simulink model "chinasim"  (R2018a)
settings: Solver=FixedStepDiscrete  StartTime=0.0  StopTime=10.0  RelTol=1e-3
InitFcn:
  | mbd_pnt_consistency_checks(bdroot(gcs));
  | t = 1
  | f = 1/t
undefined symbols (not defined in the file): B14, C10
libraries: mbd_pnt_ec_toolbox x4, dspswit3 x1
settings Model: Creator=oolonthegreat  LastModifiedBy=oolonthegreat
settings DataIOCC: ExternalInput=off  InitialState=off  SaveOutput=off  SignalLogging=off  SaveTime=off
settings OptimizationCC: DefaultParameterBehavior=Inlined  EnhancedBackFolding=on  PassReuseOutputArgsAs=Individual arguments  OptimizeBlockOrder=speed  DifferentSizesBufferReuse=on  OptimizationCustomize=off
settings DebuggingCC: InheritedTsInSrcMsg=none  SingleTaskRateTransMsg=error  ParameterTunabilityLossMsg=error  UnconnectedInputMsg=error  UnconnectedOutputMsg=error  UnconnectedLineMsg=error  UnknownTsInhSupMsg=error
settings HardwareCC: ProdBitPerPointer=32  ProdBitPerSizeT=32  ProdBitPerPtrDiffT=32  ProdLargestAtomicInteger=Long  ProdLargestAtomicFloat=Double  ProdEndianess=BigEndian  ProdWordSize=32  ProdHWDeviceType=Motorola PowerPC
settings SFSimCC: MATLABDynamicMemAlloc=off
settings RTWCC: SystemTargetFile=mbd_pnt.tlc  MakeCommand=mbd_pnt_make_rtw COPY_MDLREF_INCLUDES=0  TemplateMakefile=mbd_pnt.tmf  PostCodeGenCommand=mbd_pnt_analyzegencode(buildInfo)  Description=Model Based Design Toolbox MPC574xP Code Generation Target  GenerateReport=on  IncludeHyperlinkInReport=on  LaunchReport=on  GenerateTraceInfo=on  GenerateTraceReport=on  GenerateTraceReportSl=on  GenerateTraceReportSf=on  GenerateTraceReportEml=on
settings CodeAppCC: ForceParamTrailComments=on  IgnoreCustomStorageClasses=off  OperatorAnnotations=on  SimulinkDataObjDesc=on  SFDataObjDesc=on  InsertBlockDesc=on
settings STFCustomTargetCC: TargetLangStandard=C99 (ISO)  MultiwordLength=256  CombineOutputUpdateFcns=on  SuppressErrorStatus=on  ERTCustomFileBanners=on  SupportContinuousTime=off  SupportNonInlinedSFcns=off  RemoveResetFunc=on  MATLABClassNameForMDSCustomization=Simulink.SoftwareTarget.ERTCustomization  GRTInterface=off  SystemTargetFile=mbd_pnt.tlc
settings ERTTargetCC: TargetLangStandard=C99 (ISO)  ParMdlRefBuildCompliant=off  CompOptLevelCompliant=off  ConcurrentExecutionCompliant=off  SuppressErrorStatus=on  ModelStepFunctionPrototypeControlCompliant=off  CPPClassGenCompliant=off  UseToolchainInfoCompliant=off  InlinedParameterPlacement=NonHierarchical  ERTCustomFileTemplate=example_file_process.tlc

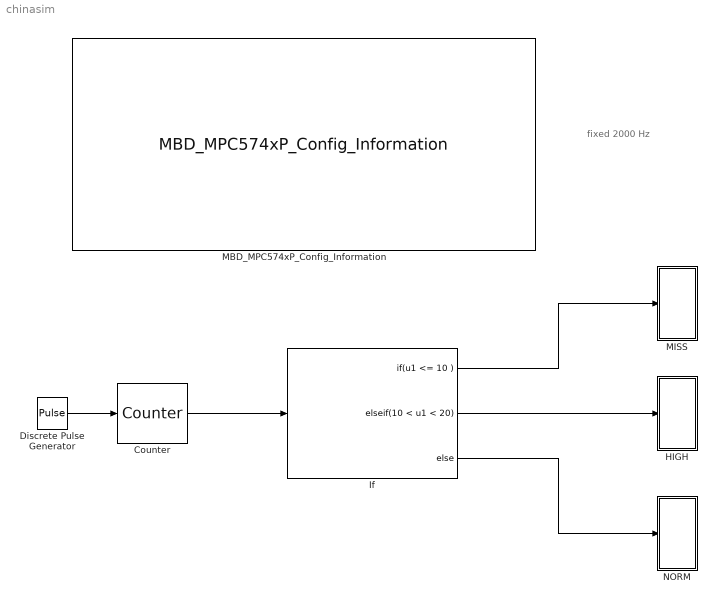
== system chinasim ==
  note: fixed 2000 Hz
  Counter : dspswit3/Counter  Direction=Up  CountEvent=Rising edge  CounterSize=User defined  MaxCount=40  InitialCount=1  Output=Count  HitValue=32  ResetInput=off  SamplesPerFrame=1  Ts=1  CntDtype=double  HitDtype=Logical
  Discrete Pulse Generator : DiscretePulseGenerator  Period=100  PulseWidth=50  SampleTime=t/10
  HIGH : Subsystem  TreatAsAtomicUnit=on
  If : If  IfExpression=u1 <= 10  ElseIfExpressions=10 < u1 < 20
  MBD_MPC574xP_Config_Information : mbd_pnt_ec_toolbox/MPC574xP/MBD_MPC574xP_Config_Information  disp_str=|  config_params=[]
      | System Clock : 200 MHz
      | Target : MPC5744P
      | Package : 144LQFP
      | XTAL Freq : 40 MHz
      | Compiler : S32 Design Studio
      | Target Type : FLASH
      | Global Interrupt Priority : 8
      | System Tick Interrupt Priority : 12
      | Freemaster : Serial1 (115200 Kbits)
      | Download Code after build : (COM5,115200)
      settings: SourceProductName=Model Based Design Toolbox for MPC574xP
  MISS : Subsystem  TreatAsAtomicUnit=on
  NORM : Subsystem  TreatAsAtomicUnit=on
  wires:
  Discrete Pulse Generator/1 -> Counter/1
  Counter/1 -> If/1
  If/1 -> MISS/Action
  If/2 -> HIGH/Action
  If/3 -> NORM/Action

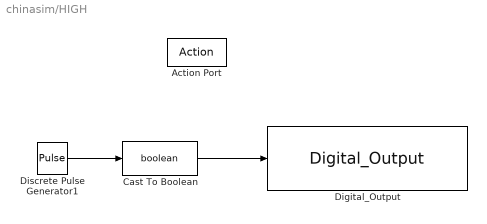
== system chinasim/HIGH ==
  Action Port : ActionPort  ActionType=elseif
  Cast To Boolean : DataTypeConversion  OutDataTypeStr=boolean
  Digital_Output : mbd_pnt_ec_toolbox/MPC574xP/Peripheral Interface Blocks/Digital_Output  gpio_outputs="42   : C10 :  [111] : [136] : [B14]"  pinNum=[111]  pcrNum=42
      settings: SourceProductName=Model Based Design Toolbox for MPC574xP
  Discrete Pulse Generator1 : DiscretePulseGenerator  Period=100  PulseWidth=50  SampleTime=t/10
  wires:
  Discrete Pulse Generator1/1 -> Cast To Boolean/1
  Cast To Boolean/1 -> Digital_Output/1

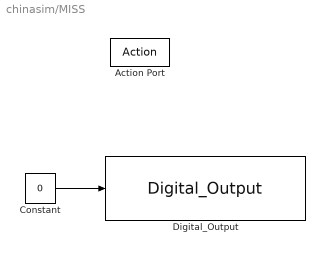
== system chinasim/MISS ==
  Action Port : ActionPort  ActionType=then
  Constant : Constant  Value=0  OutDataTypeStr=boolean
  Digital_Output : mbd_pnt_ec_toolbox/MPC574xP/Peripheral Interface Blocks/Digital_Output  gpio_outputs="42   : C10 :  [111] : [136] : [B14]"  pinNum=[111]  pcrNum=42
      settings: SourceProductName=Model Based Design Toolbox for MPC574xP
  wires:
  Constant/1 -> Digital_Output/1

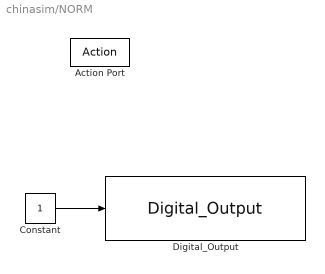
== system chinasim/NORM ==
  Action Port : ActionPort  ActionType=else
  Constant : Constant  OutDataTypeStr=boolean
  Digital_Output : mbd_pnt_ec_toolbox/MPC574xP/Peripheral Interface Blocks/Digital_Output  gpio_outputs="42   : C10 :  [111] : [136] : [B14]"  pinNum=[111]  pcrNum=42
      settings: SourceProductName=Model Based Design Toolbox for MPC574xP
  wires:
  Constant/1 -> Digital_Output/1
